simulink model "Pacemaker_3MD3_Group1"  (R2022a)
settings: Solver=FixedStepAuto  StartTime=0.0  StopTime=60  FixedStep=1e-3  RelTol=1e-3  EnableMultiTasking=on
undefined symbols (not defined in the file or in its folder): ARP, ATR_Amplitude, ATR_CMP_DETECT, ATR_Pulse_Width, ATR_Sensitivity, Hecate_delayOff, Hecate_delayOn, Hecate_HeartFail, Hecate_Mode, LRL, Mode, VENT_Amplitude, VENT_CMP_DETECT, VENT_Pulse_Width, VENT_Sensitivity, VRP
settings Model: ExtModeTrigDuration=5  Creator=akshayjacob  LastModifiedBy=fedformi_new
settings DataIOCC: SaveFormat=Structure  SaveState=on  SignalLogging=off  DSMLogging=off  StateSaveName=XT  OutputSaveName=YT
settings OptimizationCC: DefaultParameterBehavior=Inlined  EnhancedBackFolding=on  PassReuseOutputArgsAs=Individual arguments  ZeroExternalMemoryAtStartup=off  ZeroInternalMemoryAtStartup=off  MaxStackSize=64  OptimizeBlockOrder=speed  DifferentSizesBufferReuse=on  OptimizationCustomize=off  EfficientTunableParamExpr=on
settings DebuggingCC: ParameterTunabilityLossMsg=error  UnconnectedInputMsg=warning  UnconnectedOutputMsg=warning  UnconnectedLineMsg=warning
settings HardwareCC: ProdBitPerPointer=32  ProdBitPerSizeT=32  ProdBitPerPtrDiffT=32  ProdLargestAtomicInteger=Long  ProdLargestAtomicFloat=Double  ProdWordSize=32  ProdHWDeviceType=ARM Compatible->ARM Cortex
settings SFSimCC: MATLABDynamicMemAlloc=off
settings RTWCC: SystemTargetFile=ert.tlc  TemplateMakefile=ert_default_tmf  Toolchain=GNU Tools for ARM Embedded Processors  DLArmComputeVersion=19.05
settings CodeAppCC: ForceParamTrailComments=on  IgnoreCustomStorageClasses=off  OperatorAnnotations=on  SimulinkDataObjDesc=on  SFDataObjDesc=on  InsertBlockDesc=on
settings ERTTargetCC: ERTCustomFileTemplate=example_file_process.tlc

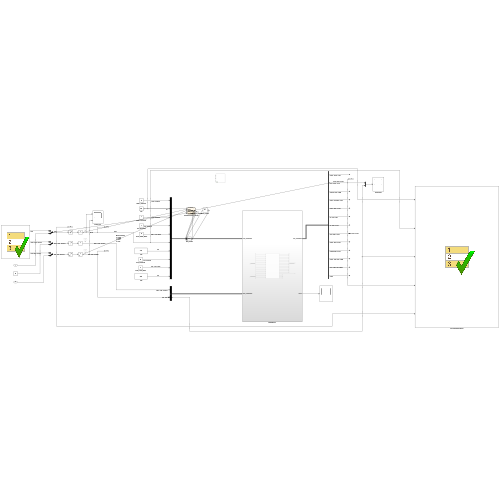
[thumbnail: Simulink's stored preview of the top-level diagram]
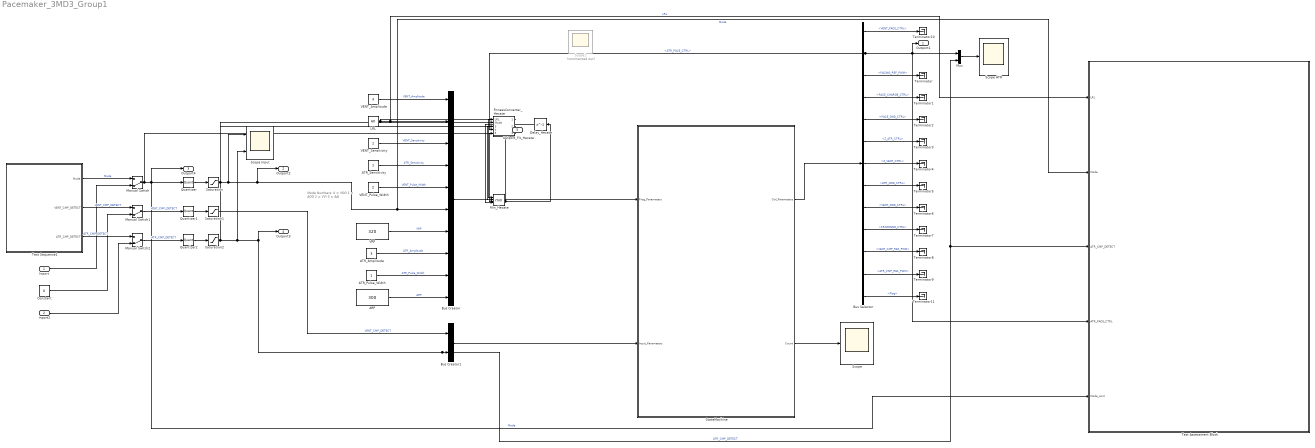
== system Pacemaker_3MD3_Group1 ==
  note: Mode Numbers:
      | 0 = VOO
      | 1 = AOO
      | 2 = VVI
      | 3 = AAI
  Inport : Inport
  Inport2 : Inport  Port=2
  ARP : Constant  Value=300
  ATR_Amplitude : Constant  Value=3
  ATR_Pulse_Width : Constant
  ATR_Sensitivity : Constant
  Bus Creator : BusCreator  Inputs=VENT_Amplitude,LRL,VENT_Sensitivity,ATR_Sensitivity,VENT_Pulse_Width,Mode,VRP,ATR_Amplitude,ATR_Pulse_Width,ARP
  Bus Creator1 : BusCreator  Inputs=VENT_CMP_DETECT,ATR_CMP_DETECT
  Bus Selector : BusSelector  OutputSignals=VENT_PACE_CTRL,ATR_PACE_CTRL,PACING_REF_PWM,PACE_CHARGE_CTRL,PACE_GND_CTRL,Z_ATR_CTRL,Z_VENT_CTRL,ATR_GND_CTRL,VENT_GND_CTRL,FRONTEND_CTRL,VENT_CMP_REF_PWM,ATR_CMP_REF_PWM,Flag
  Constant : Constant  Value=0
  Delay_Hecate : Delay  DelayLength=1  InitialCondition=Inf
  FitnessConverter_Hecate : Stateflow chart  TreatAsAtomicUnit=on
  LRL : Constant  Value=60
  Manual Switch : ManualSwitch  CurrentSetting=0
  Manual Switch1 : ManualSwitch  CurrentSetting=0
  Manual Switch2 : ManualSwitch  CurrentSetting=0
  Min_Hecate : MinMax  Inputs=4
  Mux : Mux  Inputs=2
  Quantizer : Quantizer  QuantizationInterval=1
  Quantizer1 : Quantizer  QuantizationInterval=1
  Quantizer2 : Quantizer  QuantizationInterval=1
  Saturation : Saturate  UpperLimit=3  LowerLimit=0
  Saturation1 : Saturate  UpperLimit=1  LowerLimit=0
  Saturation2 : Saturate  UpperLimit=1  LowerLimit=0
  Scope : Scope
  Scope ATR : Scope
  Scope Input : Scope  NumInputPorts=2
  Scope1 : Scope  Commented=on  NumInputPorts=3
  StateMachine : Subsystem
  Terminator{,1..11} (12 alike) : Terminator
  Test Assessment Block : Test Sequence  Tag=__SLT_ASMT__  TreatAsAtomicUnit=on
  Test Sequence1 : Test Sequence  TreatAsAtomicUnit=on
  VENT_Amplitude : Constant  Value=3
  VENT_Pulse_Width : Constant  Value=2
  VENT_Sensitivity : Constant
  VRP : Constant  Value=320
  Outport1 : Outport
  Outport2 : Outport  Port=2
  Outport4 : Outport  Port=3
  Outport3 : Outport  Port=4
  Outport_Fit_Hecate : Outport  Port=5
  wires:
  Bus Creator/1 -> StateMachine/1(Prog_Parameters)
  Bus Creator1/1 -> StateMachine/2(Input_Parameters)
  VRP/1 -> Bus Creator/7  "VRP"
  ATR_Sensitivity/1 -> Bus Creator/4  "ATR_Sensitivity"
  ATR_Pulse_Width/1 -> Bus Creator/9  "ATR_Pulse_Width"
  LRL/1 -> Test Assessment Block/1(LRL), Bus Creator/2, FitnessConverter_Hecate/1(LRL)  "LRL"
  ATR_Amplitude/1 -> Bus Creator/8  "ATR_Amplitude"
  ARP/1 -> Bus Creator/10  "ARP"
  VENT_Sensitivity/1 -> Bus Creator/3  "VENT_Sensitivity"
  VENT_Amplitude/1 -> Bus Creator/1  "VENT_Amplitude"
  VENT_Pulse_Width/1 -> Bus Creator/5  "VENT_Pulse_Width"
  Manual Switch/1 -> Outport4/1, Test Assessment Block/5(Mode_cont), Quantizer/1, FitnessConverter_Hecate/5(Mode_cont)  "Mode"
  Manual Switch1/1 -> Quantizer1/1  "VENT_CMP_DETECT"
  Manual Switch2/1 -> Quantizer2/1  "ATR_CMP_DETECT"
  Bus Selector/12 -> Terminator9/1  "<ATR_CMP_REF_PWM>"
  Bus Selector/3 -> Terminator/1  "<PACING_REF_PWM>"
  Bus Selector/7 -> Terminator4/1  "<Z_VENT_CTRL>"
  Bus Selector/10 -> Terminator7/1  "<FRONTEND_CTRL>"
  Bus Selector/8 -> Terminator5/1  "<ATR_GND_CTRL>"
  StateMachine/1(Ctrl_Parameters) -> Bus Selector/1
  Bus Selector/5 -> Terminator2/1  "<PACE_GND_CTRL>"
  Bus Selector/9 -> Terminator6/1  "<VENT_GND_CTRL>"
  Bus Selector/2 -> Test Assessment Block/4(ATR_PACE_CTRL), Mux/1, Outport1/1, FitnessConverter_Hecate/4(ATR_PACE_CTRL)  "<ATR_PACE_CTRL>"
  Bus Selector/11 -> Terminator8/1  "<VENT_CMP_REF_PWM>"
  Bus Selector/6 -> Terminator3/1  "<Z_ATR_CTRL>"
  Bus Selector/4 -> Terminator1/1  "<PACE_CHARGE_CTRL>"
  Test Sequence1/1(Mode) -> Manual Switch/1  "Mode"
  Test Sequence1/2(VENT_CMP_DETECT) -> Manual Switch1/1  "VENT_CMP_DETECT"
  Test Sequence1/3(ATR_CMP_DETECT) -> Manual Switch2/1  "ATR_CMP_DETECT"
  Inport/1 -> Manual Switch/2
  Constant/1 -> Manual Switch1/2
  Inport2/1 -> Manual Switch2/2
  Quantizer/1 -> Saturation/1
  Saturation/1 -> Scope Input/1, Outport2/1, Bus Creator/6, Test Assessment Block/2(Mode), FitnessConverter_Hecate/2(Mode)  "Mode"
  Quantizer1/1 -> Saturation1/1
  Saturation1/1 -> Bus Creator1/1  "VENT_CMP_DETECT"
  Quantizer2/1 -> Saturation2/1
  Saturation2/1 -> Scope Input/2, Outport3/1, Mux/2, Test Assessment Block/3(ATR_CMP_DETECT), Bus Creator1/2, FitnessConverter_Hecate/3(ATR_CMP_DETECT)  "ATR_CMP_DETECT"
  Mux/1 -> Scope ATR/1
  StateMachine/2(Count) -> Scope/1
  Bus Selector/1 -> Terminator10/1  "<VENT_PACE_CTRL>"
  Bus Selector/13 -> Terminator11/1  "<Flag>"
  FitnessConverter_Hecate/1(fitness_1) -> Min_Hecate/1
  FitnessConverter_Hecate/2(fitness_2) -> Min_Hecate/2
  FitnessConverter_Hecate/3(fitness_3) -> Min_Hecate/3
  Min_Hecate/1 -> Delay_Hecate/1, Outport_Fit_Hecate/1
  Delay_Hecate/1 -> Min_Hecate/4

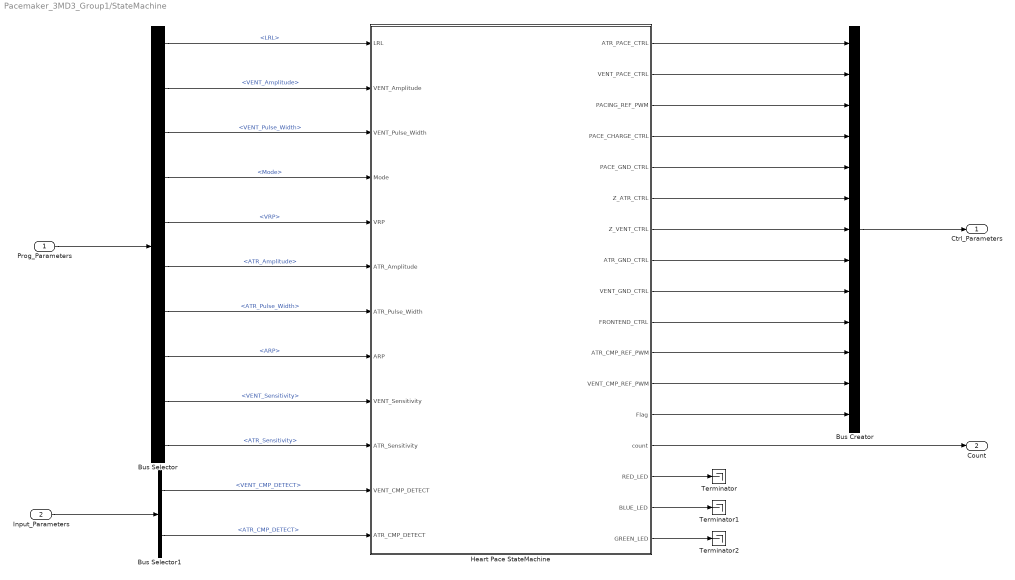
== system Pacemaker_3MD3_Group1/StateMachine ==
  Prog_Parameters : Inport
  Input_Parameters : Inport  Port=2
  Bus Creator : BusCreator  Inputs=13
  Bus Selector : BusSelector  OutputSignals=LRL,VENT_Amplitude,VENT_Pulse_Width,Mode,VRP,ATR_Amplitude,ATR_Pulse_Width,ARP,VENT_Sensitivity,ATR_Sensitivity
  Bus Selector1 : BusSelector  OutputSignals=VENT_CMP_DETECT,ATR_CMP_DETECT
  Heart Pace StateMachine : Stateflow chart  TreatAsAtomicUnit=on
      settings: PortSchema="{\"entries\":[{\"content\":{\"sides\":[{\"content\":{\"connectorIds\":[\"In1\",\"In2\",\"In3\",\"In4\",\"In5\",\"In6\",\"In7\",\"In8\",\"In9\",\"In10\",\"In11\",\"In12\"]},\"type\":\"ConnectorPlacement.EquallySpacedRectSide\",\"uuid\":\"078f44e2-9792-46c6-9fab-c05fe0916fc5\"},{\"content\":{\"connectorIds\":[\"Out1\",\"Out2\",\"Out3\",\"Out4\",\"Out5\",\"Out6\",\"Out7\",\"Out8\",\"Out9\",\"Out10\",\"Out14\",\"Out15\",\"Out16\",\"Out17\",\"Out11\",\"Out12\",\"Out13\"],\"side\":\"RIGHT\"},\"type\":\"ConnectorPlacement.EquallySpacedRectSide\",\"uuid\":\"2df68980-2ea6-42d1-b726-b24978220bfa\"},{\"content\":{\"connectorIds\":[],\"side\":\"TOP\"},\"type\":\"ConnectorPlacement.EquallySpacedRectSide\",\"uuid\":\"4f99418a-e276-4e4c-8fb0-96ffb017fecf\"}]},\"type\":\"ConnectorPlacement.EquallySpacedConnector\",\"uuid\":\"ac4267e7-732c-486f-b9a5-28cca0f40ec4\"}],\"packageUris\":[\"http://schema.mathworks.com/mf0/Connector/R2020b\"],\"version\":\"1.0\"}"
  Terminator : Terminator
  Terminator1 : Terminator
  Terminator2 : Terminator
  Ctrl_Parameters : Outport
  Count : Outport  Port=2
  wires:
  Prog_Parameters/1 -> Bus Selector/1
  Bus Selector/1 -> Heart Pace StateMachine/1(LRL)  "<LRL>"
  Bus Selector/2 -> Heart Pace StateMachine/2(VENT_Amplitude)  "<VENT_Amplitude>"
  Bus Selector/3 -> Heart Pace StateMachine/3(VENT_Pulse_Width)  "<VENT_Pulse_Width>"
  Bus Selector/4 -> Heart Pace StateMachine/4(Mode)  "<Mode>"
  Heart Pace StateMachine/1(ATR_PACE_CTRL) -> Bus Creator/1
  Heart Pace StateMachine/2(VENT_PACE_CTRL) -> Bus Creator/2
  Bus Creator/1 -> Ctrl_Parameters/1
  Heart Pace StateMachine/3(PACING_REF_PWM) -> Bus Creator/3
  Heart Pace StateMachine/4(PACE_CHARGE_CTRL) -> Bus Creator/4
  Heart Pace StateMachine/5(PACE_GND_CTRL) -> Bus Creator/5
  Heart Pace StateMachine/6(Z_ATR_CTRL) -> Bus Creator/6
  Heart Pace StateMachine/7(Z_VENT_CTRL) -> Bus Creator/7
  Heart Pace StateMachine/8(ATR_GND_CTRL) -> Bus Creator/8
  Heart Pace StateMachine/9(VENT_GND_CTRL) -> Bus Creator/9
  Heart Pace StateMachine/10(FRONTEND_CTRL) -> Bus Creator/10
  Input_Parameters/1 -> Bus Selector1/1
  Bus Selector1/1 -> Heart Pace StateMachine/11(VENT_CMP_DETECT)  "<VENT_CMP_DETECT>"
  Bus Selector1/2 -> Heart Pace StateMachine/12(ATR_CMP_DETECT)  "<ATR_CMP_DETECT>"
  Bus Selector/6 -> Heart Pace StateMachine/6(ATR_Amplitude)  "<ATR_Amplitude>"
  Bus Selector/7 -> Heart Pace StateMachine/7(ATR_Pulse_Width)  "<ATR_Pulse_Width>"
  Bus Selector/8 -> Heart Pace StateMachine/8(ARP)  "<ARP>"
  Bus Selector/9 -> Heart Pace StateMachine/9(VENT_Sensitivity)  "<VENT_Sensitivity>"
  Bus Selector/10 -> Heart Pace StateMachine/10(ATR_Sensitivity)  "<ATR_Sensitivity>"
  Heart Pace StateMachine/14(ATR_CMP_REF_PWM) -> Bus Creator/11
  Heart Pace StateMachine/15(VENT_CMP_REF_PWM) -> Bus Creator/12
  Bus Selector/5 -> Heart Pace StateMachine/5(VRP)  "<VRP>"
  Heart Pace StateMachine/16(Flag) -> Bus Creator/13
  Heart Pace StateMachine/11(RED_LED) -> Terminator/1
  Heart Pace StateMachine/12(BLUE_LED) -> Terminator1/1
  Heart Pace StateMachine/13(GREEN_LED) -> Terminator2/1
  Heart Pace StateMachine/17(count) -> Count/1

== stateflow chart Pacemaker_3MD3_Group1/Test Assessment Block ==
  state Partial
    state Mode_selection
      state Mode_3
        state Sensing
        state Heartbeat
          verify(true)
        state No_heartbeat
          verify(false)
        (junction 689) -> (junction 660)
        (default) -> Sensing
        (junction 660) -> Sensing
        Sensing -> (junction 670) [order 2] : [
            | et > 60/LRL
            | ]
        (junction 670) -> (junction 652)
        Sensing -> Heartbeat [order 1] : [
            | ATR_CMP_DETECT == true || ATR_PACE_CTRL == true
            | ]
        Heartbeat -> Sensing : [
            | true
            | ]
        (junction 652) -> No_heartbeat
        No_heartbeat -> (junction 689) : [
            | ATR_CMP_DETECT == true || ATR_PACE_CTRL == true
            | ]
      state Else
        verify(Mode_cont <= 3.5)
      (junction 637) -> (junction 640) [order 2]
      (junction 627) -> (junction 636) [order 2]
      (default) -> (junction 627)
      Mode_selection -> (junction 627)
      (junction 627) -> (junction 628) [order 1] : [(Mode == 3)
          | ]
      (junction 628) -> Mode_3 [order 1] : [~in(Partial.Mode_selection.Mode_3)]
      (junction 628) -> (junction 631) [order 2]
      (junction 636) -> (junction 637)
      (junction 637) -> Else [order 1] : [~in(Partial.Mode_selection.Else)]
    (default) -> Mode_selection
  (default) -> Partial : {assert(Active_Scenario_Index == 1,'The value of Scenario Parameter ''Active_Scenario_Index'' is not valid. Use the index of the scenario to specify it.')}
  data: LRL input double size=[1]; Mode input double size=[1]; ATR_CMP_DETECT input size=[1, 1]; ATR_PACE_CTRL input double size=[1]; Active_Scenario_Index parameter =1; Mode_cont input

== stateflow chart Pacemaker_3MD3_Group1/Test Sequence1 ==
  settings: updateMethod=DISCRETE  sampleTime=0.001
  state AAI_Mode_3
    Mode=Hecate_Mode;
    VENT_CMP_DETECT=false;
    state AAI_Mode_3_OFF
      ATR_CMP_DETECT=false;
    state AAI_Mode_3_ON
      ATR_CMP_DETECT=true;
    (default) -> AAI_Mode_3_OFF
    AAI_Mode_3_OFF -> AAI_Mode_3_ON : [
        | after(2+Hecate_delayOn,sec)
        | ]
    AAI_Mode_3_ON -> AAI_Mode_3_OFF : [
        | after(0.05+Hecate_delayOff,sec)
        | ]
  state END
    ATR_CMP_DETECT=false;
  (default) -> AAI_Mode_3
  AAI_Mode_3 -> END : [
      | after(Hecate_HeartFail,sec)
      | ]
  data: Mode output double size=[1]; VENT_CMP_DETECT output boolean size=[1, 1]; ATR_CMP_DETECT output boolean size=[1, 1]; Hecate_HeartFail parameter; Hecate_delayOn parameter; Hecate_delayOff parameter; Hecate_Mode parameter

== stateflow chart Pacemaker_3MD3_Group1/FitnessConverter_Hecate ==
  state Mode_selection
    fitness_1 = Inf;
    fitness_2 = Inf;
    fitness_3 = Inf;
    state Mode_3
      fitness_1 = Inf;
      fitness_2 = Inf;
      fitness_3 = Inf;
      state Sensing
        fitness_1 = Inf;
        fitness_2 = Inf;
        fitness_3 = Inf;
      state Heartbeat
        fitness_1 = 1;
        fitness_2 = Inf;
        fitness_3 = Inf;
      state No_heartbeat
        fitness_1 = Inf;
        fitness_2 = -1;
        fitness_3 = Inf;
      (default) -> Sensing
      No_heartbeat -> Sensing : [ATR_CMP_DETECT == true || ATR_PACE_CTRL == true]
      Heartbeat -> Sensing : [true]
      Sensing -> Heartbeat [order 1] : [ATR_CMP_DETECT == true || ATR_PACE_CTRL == true]
      Sensing -> No_heartbeat [order 2] : [et > 60/LRL]
    state Else
      fitness_1 = Inf;
      fitness_2 = Inf;
      fitness_3 = 3.5-(Mode_cont);
    (default) -> (junction 4)
    Else -> (junction 4) : [((Mode == 3))]
    (junction 4) -> Mode_3 [order 1] : [(Mode == 3)]
    (junction 4) -> Else [order 2] : []
    Mode_3 -> (junction 4) : [~((Mode == 3))]
  (default) -> Mode_selection
  data: LRL input; Mode input; ATR_CMP_DETECT input; ATR_PACE_CTRL input; Mode_cont input; fitness_1 output; fitness_2 output; fitness_3 output

== stateflow chart Pacemaker_3MD3_Group1/StateMachine/Heart Pace StateMachine ==
  state VOO_ChargingState
    entry:
    ATR_PACE_CTRL = 0;
    VENT_PACE_CTRL = 0;
    PACING_REF_PWM = VENT_Amplitude/5*100;
    PACE_CHARGE_CTRL = 1;
    PACE_GND_CTRL = 1;
    Z_ATR_CTRL = 0;
    Z_VENT_CTRL = 0;
    ATR_GND_CTRL = 0;
    VENT_GND_CTRL = 1;
    BLUE_LED = 0;
    RED_LED = 1;
  state VOO_Pacing
    entry:
    PACE_CHARGE_CTRL = 0;
    PACE_GND_CTRL = 1;
    ATR_GND_CTRL = 0;
    ATR_PACE_CTRL = 0;
    Z_ATR_CTRL = 0;
    Z_VENT_CTRL =0;
    VENT_PACE_CTRL = 1;
    VENT_GND_CTRL = 0;
    PACING_REF_PWM = VENT_Amplitude/5*100;
    BLUE_LED=1;
    RED_LED=0;
  state AOO_ChargingState
    entry:
    ATR_PACE_CTRL = 0;
    VENT_PACE_CTRL = 0;
    PACING_REF_PWM = ATR_Amplitude/5*100;
    PACE_CHARGE_CTRL = 1;
    PACE_GND_CTRL = 1;
    Z_ATR_CTRL = 0;
    Z_VENT_CTRL = 0;
    ATR_GND_CTRL = 1;
    VENT_GND_CTRL = 0;
    BLUE_LED = 0;
    RED_LED = 1;
  state AOO_Pacing
    entry:
    PACE_CHARGE_CTRL = 0;
    PACE_GND_CTRL = 1;
    ATR_GND_CTRL = 0;
    ATR_PACE_CTRL = 1;
    Z_ATR_CTRL = 0;
    Z_VENT_CTRL =0;
    VENT_PACE_CTRL = 0;
    VENT_GND_CTRL = 0;
    PACING_REF_PWM = ATR_Amplitude/5*100;
    BLUE_LED=1;
    RED_LED=0;
  state MAIN
    entry:
    PACE_CHARGE_CTRL = 0;
    VENT_PACE_CTRL = 0;
    ATR_PACE_CTRL = 0;
    PACE_GND_CTRL = 0;
    ATR_GND_CTRL = 0;
    VENT_GND_CTRL = 0;
    Z_ATR_CTRL = 0;
    Z_VENT_CTRL = 0;
    FRONTEND_CTRL = 0;
    RED_LED = 0;
    BLUE_LED=0;
    Flag = 0;
    count = 0;
  state VVI_Sensing
    entry:
    BLUE_LED = 0;
    RED_LED = 0;
    GREEN_LED = 1;
    FRONTEND_CTRL = 1;
    Flag = 0;
  state VVI_Refactory
    entry:
    ATR_PACE_CTRL = 0;
    VENT_PACE_CTRL = 0;
    PACING_REF_PWM = VENT_Amplitude/5*100;
    PACE_CHARGE_CTRL = 1;
    PACE_GND_CTRL = 1;
    Z_ATR_CTRL = 0;
    Z_VENT_CTRL = 0;
    ATR_GND_CTRL = 0;
    VENT_GND_CTRL = 1;
    FRONTEND_CTRL = 1;
    VENT_CMP_REF_PWM = VENT_Sensitivity/5*100;
    BLUE_LED = 0;
    RED_LED = 1;
    GREEN_LED = 0;
  state VVI_Pacing
    entry:
    FRONTEND_CTRL = 0;
    PACE_CHARGE_CTRL = 0;
    PACE_GND_CTRL = 1;
    ATR_GND_CTRL = 0;
    ATR_PACE_CTRL = 0;
    Z_ATR_CTRL = 0;
    Z_VENT_CTRL =0;
    VENT_PACE_CTRL = 1;
    VENT_GND_CTRL = 0;
    PACING_REF_PWM = VENT_Amplitude/5*100;
    BLUE_LED = 1;
    RED_LED = 0;
    GREEN_LED = 0;
    Flag = 1;
  state AAI_Sensing
    entry:
    BLUE_LED = 0;
    RED_LED = 0;
    GREEN_LED = 1;
    Flag = 0;
  note: Subtract PW from this based on previous event
      | -sense heart rate: dont (no pulsewith done by pacemaker)
      | -pulsed rate: subtract PW
      |  vrp-(pulsewith*flag)
  state AAI_Refactory
    entry:
    ATR_PACE_CTRL = 0;
    VENT_PACE_CTRL = 0;
    PACING_REF_PWM = ATR_Amplitude/5*100;
    PACE_CHARGE_CTRL = 1;
    PACE_GND_CTRL = 1;
    Z_ATR_CTRL = 0;
    Z_VENT_CTRL = 0;
    ATR_GND_CTRL = 1;
    VENT_GND_CTRL = 0;
    FRONTEND_CTRL = 1;
    ATR_CMP_REF_PWM= ATR_Sensitivity/5*100;
    BLUE_LED = 0;
    RED_LED = 1;
    GREEN_LED = 1;
  state AAI_Pacing
    entry:
    FRONTEND_CTRL = 0;
    PACE_CHARGE_CTRL = 0;
    PACE_GND_CTRL = 1;
    ATR_GND_CTRL = 0;
    ATR_PACE_CTRL = 1;
    Z_ATR_CTRL = 0;
    Z_VENT_CTRL =0;
    VENT_PACE_CTRL = 0;
    VENT_GND_CTRL = 0;
    PACING_REF_PWM = ATR_Amplitude/5*100;
    BLUE_LED = 1;
    RED_LED = 0;
    GREEN_LED = 0;
    Flag = 1;
    count = count+1;
  state AAI_Failure
    count = 0;
  VOO_ChargingState -> VOO_Pacing : after((60000/LRL) - VENT_Pulse_Width,msec)
  MAIN -> VOO_ChargingState [order 1] : [Mode == 0]
  VOO_Pacing -> VOO_ChargingState : after(VENT_Pulse_Width, msec)
  (default) -> MAIN
  AOO_ChargingState -> AOO_Pacing : after((60000/LRL) - ATR_Pulse_Width,msec)
  MAIN -> AOO_ChargingState [order 4] : [Mode == 1]
  AOO_Pacing -> AOO_ChargingState : after(ATR_Pulse_Width, msec)
  MAIN -> VVI_Refactory [order 2] : [Mode == 2]
  MAIN -> AAI_Refactory [order 3] : [Mode==3]
  VVI_Refactory -> VVI_Sensing : after(VRP - (VENT_Pulse_Width * Flag),msec)
  VVI_Sensing -> VVI_Pacing [order 2] : after(60000/LRL - VRP, msec)
  VVI_Sensing -> VVI_Refactory [order 1] : [(VENT_CMP_DETECT == 1)]
  VVI_Pacing -> VVI_Refactory : after(VENT_Pulse_Width,msec)
  AAI_Refactory -> AAI_Sensing : after(ARP  - (ATR_Pulse_Width * Flag),msec)
  AAI_Sensing -> AAI_Pacing [order 3] : after(60000/LRL - ARP, msec)
  AAI_Sensing -> AAI_Refactory [order 1] : [ATR_CMP_DETECT >= 1]
  AAI_Sensing -> AAI_Failure [order 2] : [count >= 55]
  AAI_Pacing -> AAI_Refactory : after(ATR_Pulse_Width,msec)
  AAI_Failure -> AAI_Refactory : after(ATR_Pulse_Width,msec)
  data: LRL input; VENT_Amplitude input; VENT_Pulse_Width input; Mode input; ATR_PACE_CTRL output; VENT_PACE_CTRL output; PACING_REF_PWM output; PACE_CHARGE_CTRL output; PACE_GND_CTRL output; Z_ATR_CTRL output; Z_VENT_CTRL output; ATR_GND_CTRL output; VENT_GND_CTRL output; FRONTEND_CTRL output; RED_LED output =0; BLUE_LED output; VRP input; ATR_Amplitude input; ATR_Pulse_Width input; ARP input; VENT_Sensitivity input; ATR_Sensitivity input; GREEN_LED output; VENT_CMP_DETECT input; ATR_CMP_DETECT input; ATR_CMP_REF_PWM output; VENT_CMP_REF_PWM output; Flag output; count output double =0
